simulink model "gm_sine_gen"  (R2024b)
settings: Solver=VariableStepAuto  StartTime=0.0  StopTime=10/200e3  RelTol=1e-3
InitFcn:
  | f_sim=1/5e6;
libraries: dspsrcs4 x3
settings Model: Creator=angro  LastModifiedBy=angro
settings OptimizationCC: BlockReduction=off  ConditionallyExecuteInputs=off
settings DebuggingCC: InheritedTsInSrcMsg=none

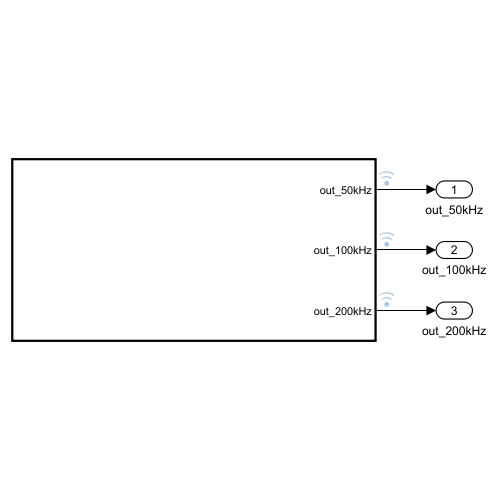
[thumbnail: Simulink's stored preview of the top-level diagram]
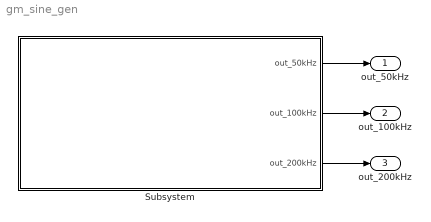
== system gm_sine_gen ==
  Subsystem : Subsystem  TreatAsAtomicUnit=on  SystemSampleTime=f_sim
  out_50kHz : Outport
  out_100kHz : Outport  Port=2
  out_200kHz : Outport  Port=3
  wires:
  Subsystem/3(out_200kHz) -> out_200kHz/1
  Subsystem/2(out_100kHz) -> out_100kHz/1
  Subsystem/1(out_50kHz) -> out_50kHz/1

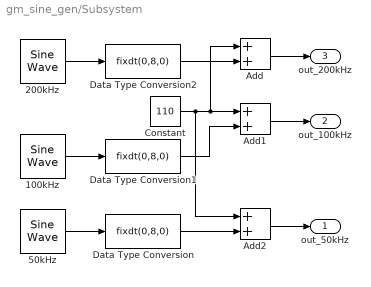
== system gm_sine_gen/Subsystem ==
  100kHz : dspsrcs4/Sine Wave  Amplitude=100  Frequency=100e3  Phase=0  SampleMode=Discrete  OutComplex=Real  CompMethod=Table lookup  TableSize=Speed  SampleTime=f_sim  SamplesPerFrame=1  ResetState=Restart at time zero  OutputFrames=off  dataType=Fixed-point  wordLen=16  udDataType=sfix(16)  fracBitsMode=User-defined  numFracBits=0  OutDataTypeStr=fixdt(1,16,0)  LastOutDataTypeStr=fixdt(1,16,0)
  200kHz : dspsrcs4/Sine Wave  Amplitude=100  Frequency=200e3  Phase=0  SampleMode=Discrete  OutComplex=Real  CompMethod=Table lookup  TableSize=Speed  SampleTime=f_sim  SamplesPerFrame=1  ResetState=Restart at time zero  OutputFrames=off  dataType=Fixed-point  wordLen=16  udDataType=sfix(16)  fracBitsMode=User-defined  numFracBits=0  OutDataTypeStr=fixdt(1,16,0)  LastOutDataTypeStr=fixdt(1,16,0)
  50kHz : dspsrcs4/Sine Wave  Amplitude=100  Frequency=50e3  Phase=0  SampleMode=Discrete  OutComplex=Real  CompMethod=Table lookup  TableSize=Speed  SampleTime=f_sim  SamplesPerFrame=1  ResetState=Restart at time zero  OutputFrames=off  dataType=Fixed-point  wordLen=16  udDataType=sfix(16)  fracBitsMode=User-defined  numFracBits=0  OutDataTypeStr=fixdt(1,16,0)  LastOutDataTypeStr=fixdt(1,16,0)
  Add : Sum
  Add1 : Sum
  Add2 : Sum
  Constant : Constant  Value=110  OutDataTypeStr=fixdt(0,8,0)
  Data Type Conversion : DataTypeConversion  OutDataTypeStr=fixdt(0,8,0)  SaturateOnIntegerOverflow=off  RndMeth=Floor
  Data Type Conversion1 : DataTypeConversion  OutDataTypeStr=fixdt(0,8,0)  SaturateOnIntegerOverflow=off  RndMeth=Floor
  Data Type Conversion2 : DataTypeConversion  OutDataTypeStr=fixdt(0,8,0)  SaturateOnIntegerOverflow=off  RndMeth=Floor
  out_50kHz : Outport
  out_100kHz : Outport  Port=2
  out_200kHz : Outport  Port=3
  wires:
  Add2/1 -> out_50kHz/1
  Add1/1 -> out_100kHz/1
  Data Type Conversion/1 -> Add2/2
  Add/1 -> out_200kHz/1
  Data Type Conversion1/1 -> Add1/2
  Constant/1 -> Add2/1, Add1/1, Add/1
  Data Type Conversion2/1 -> Add/2
  50kHz/1 -> Data Type Conversion/1
  100kHz/1 -> Data Type Conversion1/1
  200kHz/1 -> Data Type Conversion2/1
